simulink model "mlf_decoder"  (R2015b)
settings: Solver=FixedStepDiscrete  SolverMode=SingleTasking  StartTime=0.0  StopTime=100  RelTol=1e-3
libraries: hdlsllib x2, simulink x1
settings Model: Creator=at-mt  LastModifiedBy=amatsumo
settings DataIOCC: SaveFormat=Array  SignalLoggingSaveFormat=ModelDataLogs  SaveOutput=off  SignalLogging=off  SaveTime=off
settings OptimizationCC: BlockReduction=off  ConditionallyExecuteInputs=off  DefaultParameterBehavior=Inlined  ExpressionDepthLimit=2147483647
settings DebuggingCC: AlgebraicLoopMsg=error  UnderspecifiedInitializationDetection=Classic  MergeDetectMultiDrivingBlocksExec=none  SolverPrmCheckMsg=warning  SingleTaskRateTransMsg=error  FcnCallInpInsideContextMsg=UseLocalSettings  StateNameClashWarn=warning
settings HardwareCC: ProdBitPerPointer=32  ProdLargestAtomicFloat=None  ProdIntDivRoundTo=Undefined  ProdEndianess=Unspecified  ProdWordSize=32  ProdHWDeviceType=ASIC/FPGA->ASIC/FPGA  ProdEqTarget=off
settings GRTTargetCC: GeneratePreprocessorConditionals=Disable all  CombineOutputUpdateFcns=off  GRTInterface=on
settings ConfigComp: CovModelRefEnable=Off  CovSFcnEnable=off

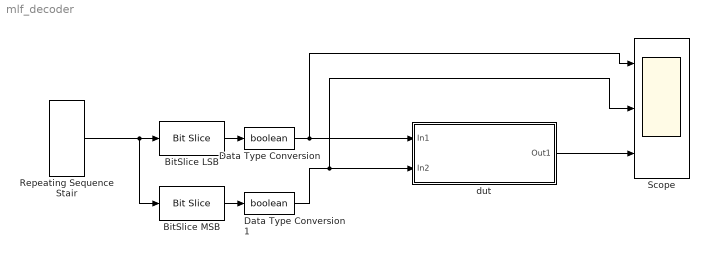
== system mlf_decoder ==
  BitSlice LSB : hdlsllib/HDL Operations/Bit Slice  lidx=0  ridx=0
  BitSlice MSB : hdlsllib/HDL Operations/Bit Slice  lidx=1  ridx=1
  Data Type Conversion : DataTypeConversion  OutDataTypeStr=boolean
  Data Type Conversion1 : DataTypeConversion  OutDataTypeStr=boolean
  Repeating Sequence Stair : simulink/Sources/Repeating Sequence Stair  OutValues=[0 1 2 1 2 0 2 1 0 1 1].'  tsamp=-1  OutMin=[]  OutMax=[]  OutDataTypeStr=fixdt(0,2,0)  OutputDataTypeScalingMode=Specify via dialog  OutDataType=fixdt(0,2,0)  ConRadixGroup=Best Precision: Vector-wise  OutScaling=[]
  Scope : Scope  NumInputPorts=3
  dut : Subsystem
  wires:
  Repeating Sequence Stair/1 -> BitSlice LSB/1, BitSlice MSB/1
  BitSlice LSB/1 -> Data Type Conversion/1
  BitSlice MSB/1 -> Data Type Conversion1/1
  dut/1(Out1) -> Scope/3
  Data Type Conversion/1 -> Scope/1, dut/1(In1)
  Data Type Conversion1/1 -> Scope/2, dut/2(In2)

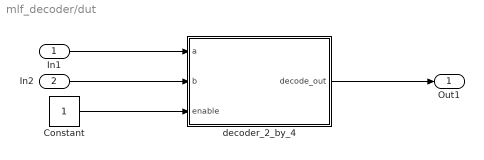
== system mlf_decoder/dut ==
  In1 : Inport
  In2 : Inport  Port=2
  Constant : Constant  OutDataTypeStr=boolean
  decoder_2_by_4 : MATLAB Function  TreatAsAtomicUnit=on
  Out1 : Outport
  wires:
  Constant/1 -> decoder_2_by_4/3(enable)
  In1/1 -> decoder_2_by_4/1(a)
  In2/1 -> decoder_2_by_4/2(b)
  decoder_2_by_4/1(decode_out) -> Out1/1

== matlab function mlf_decoder/dut/decoder_2_by_4 ==
  settings: fimath=|
      | fimath(...
      | 'RoundMode', 'floor',...
      | 'OverflowMode', 'wrap',...
      | 'ProductMode', 'FullPrecision', 'ProductWordLength', 32,...
      | 'SumMode', 'FullPrecision', 'SumWordLength', 32,...
      | 'CastBeforeSum', true)
  data: a input boolean; decode_out output fixdt(0,4,0) size=1; b input boolean; enable input boolean
function decode_out  = fcn(a, b, enable)

% 2 by 4 decoder circuit.

result_nt = numerictype(0,4,0);
result_fm = fimath('OverflowMode', 'wrap', 'RoundMode', 'floor');
decode_out = fi(0, result_nt, result_fm);

a_bar = ~a;
b_bar = ~b;

% compute bit0
decode_out = bitset(decode_out, 1, ~(enable & a_bar & b_bar));
% compute bit1
decode_out = bitset(decode_out, 2, ~(enable & a_bar & b));
% compute bit2
decode_out = bitset(decode_out, 3, ~(enable & a & b_bar));
% compute bit3
decode_out = bitset(decode_out, 4, ~(enable & a & b));
